simulink model "RemoteMicrogrid"  (R2025a)
settings: Solver=FixedStepAuto  StartTime=0.0  StopTime=8  FixedStep=Ts  MaxStep=1e-3  RelTol=1e-3
PreLoadFcn:
  | RemoteMicrogridInputData
undefined symbols (not defined in the file): BESS, ControlRoom, DiscIntNeverNeededParam, Grid, Load, Machine, Microgrid, MicrogridStatus, PV, relay1, T_on, Ts
libraries: ee_lib x53, fl_lib x39, eeGeneralControl x30, simulink x30, nesl_utility x26, nesl_utility_internal x19, slpidlib x7, eeTransforms x5, eeRmsMeasurement x4, eeTotalHarmonicDistorsion x4, batteryecm_lib x2, simulink_extras x2
(part 1 of 6)
CloseFcn:
  | figure1 = findobj('Type', 'figure', 'Name','h1_remote_microgrid');
  | figure2 = findobj('Type', 'figure', 'Name','h2_remote_microgrid');
  | figure3 = findobj('Type', 'figure', 'Name','h2a_remote_microgrid');
  | figure4 = findobj('Type', 'figure', 'Name','h3_remote_microgrid');
  | figure5 = findobj('Type', 'figure', 'Name','h4_remote_microgrid');
  | close(figure1);
  | close(figure2);
  | close(figure3);
  | close(figure4);
  | close(figure5);
  | clear figure1 figure2 figure3 figure4 figure5
  | clear BESS closedLoop controller currentLoopPole
  | clear fsw_V geometricMean grid Grid inverter KI_PVPLL
  | clear KP_PVPLL logsout_remote_microgrid
  | clear Microgrid PrimaryreactancePV PrimaryresistancePV
  | clear remainingPowerPerString SecondaryreactancePV
  | clear SecondaryresistancePV sensor simlog_remote_microgrid
  | clear simulation solarPanel solarPlant TransformerPrimaryVoltagePV
  | clear TransformerRatingPV TransformerSecondaryVoltagePV
  | clear Ts Ts_V Solar logsout_remote_microgrid simlog_remote_microgrid
  | clear caseNum ControlRoom Load Machine tStart tStop
  | clear transformer_lv transformer_hv transformer_VA
  | clear transformer_winding_resistance transformer_winding_lekage_reactance
  | clear transformer_zero_sequence_reactance I_max_pu Vdc C L KV_base_new
  | clear MVA_base_new z_base n_series_cell_panel n_parallel_strings_panel
  | clear n_series_panels_per_string n_parallel_strings t_sensor
  | clear Kp_ic Ki_ic Kd Kp_v Ki_v Kd_v Vdc_base
  | clear Kp_pll Ki_pll
  | clear diode_saturation_current solar_generated_current_AM
  | clear quality_factor_i quality_factor_j Solar_cell.series_resistance
  | clear parallel_resistance temp_cofficient Eg temparature_exponent_Is1
  | clear temparature_exponent_Is2 temparature_exponent_Rs temparature_exponent_Rp
  | clear measurement_temperature device_temperature
  | clear PV Solar_cell T_on
  | clear BESSCost1 BESSCost2 BESSCost3 BESSCost4 BESSCost5 BESSKVAs1 BESSKVAs2
  | clear BESSKVAs3 BESSKVAs4 BESSKVAs5 Diesel_cost_s1 Diesel_cost_s1_yr Diesel_cost_s2
  | clear Diesel_cost_s2_yr Diesel_cost_s3 Diesel_cost_s3_yr Diesel_cost_s4 Diesel_cost_s4_yr
  | clear Diesel_cost_s5 Diesel_cost_s5_yr diesel_litre_USD Diesel_loading_100percent
  | clear Diesel_loading_25percent Diesel_loading_50percent Diesel_loading_75percent
  | clear Diesel_s1 Diesel_s2 Diesel_s3 Diesel_s4 Diesel_s5 DieselKVAs1 DieselKVAs2
  | clear DieselKVAs3 DieselKVAs4 DieselKVAs5 frequencyLimit logsout1 logsout2 logsout3
  | clear logsout4 logsout_activeloss1 logsout_activeloss2 logsout_activeloss3
  | clear logsout_activeloss4 logsout_freqmax1 logsout_freqmax2 logsout_freqmax3
  | clear logsout_freqmax4 logsout_freqmin1 logsout_freqmin2 logsout_freqmin3 logsout_freqmin4
  | clear logsout_LoadTHD1 logsout_LoadTHD2 logsout_LoadTHD3 logsout_LoadTHD4
  | clear logsout_MaxLoadVoltage1 logsout_MaxLoadVoltage2 logsout_MaxLoadVoltage3
  | clear logsout_MaxLoadVoltage4 logsout_MinLoadVoltage1 logsout_MinLoadVoltage2
  | clear logsout_MinLoadVoltage3 logsout_MinLoadVoltage4 logsout_PCCTHD1 logsout_PCCTHD2
  | clear logsout_PCCTHD3 logsout_PCCTHD4 logsout_reactiveloss1 logsout_reactiveloss2
  | clear logsout_reactiveloss3 logsout_reactiveloss4 logsout_volmax1 logsout_volmax2
  | clear logsout_volmax3 logsout_volmax4 logsout_volmin1 logsout_volmin2 logsout_volmin3
  | clear logsout_volmin4 Micorgrid TotalCost1 TotalCost2 TotalCost3 TotalCost4 TotalCost5
  | clear voltageLimit xlim xticks
Description:
  | Copyright 2022 - 2023 The MathWorks, Inc.
settings Model: SimulationMode=accelerator  NumberOfSteps=10  Creator=The MathWorks, Inc.  LastModifiedBy=skota
settings SolverCC: ZeroCrossAlgorithm=Adaptive  AlgebraicLoopSolver=TrustRegion
settings DataIOCC: ExternalInput=getinputstruct(op)  InitialState=getstatestruct(op)  SaveOutput=off  DSMLogging=off  SaveTime=off  SignalLoggingName=logsout_RemoteMicrogrid  OutputTimes=[0:1.1*3*Voc/(1*2000):1.1*3*Voc/1]  ReturnWorkspaceOutputsName=simoutData
settings OptimizationCC: ReuseModelBlockBuffer=off
settings DebuggingCC: UnconnectedInputMsg=warning  UnconnectedOutputMsg=warning  UnconnectedLineMsg=warning  StateNameClashWarn=warning  ArithmeticOperatorsInVariantConditions=warning
settings HardwareCC: ProdBitPerPointer=32.0  ProdBitPerSizeT=32.0  ProdBitPerPtrDiffT=32.0  ProdWordSize=32.0  ProdHWDeviceType=Intel->x86-32 (Windows32)
settings ModelReferenceCC: PropagateSignalLabelsOutOfModel=off
settings SFSimCC: SFSimEcho=off  SimCtrlC=off  CustomCodeUndefinedFunction=UseInterfaceOnly
settings RTWCC: Toolchain=MinGW64 | gmake (64-bit Windows)  GPUComputeCapability=3.5  DLArmComputeVersion=19.05
settings CodeAppCC: StateflowObjectComments=on
settings SimscapeCC: SimscapeNominalValues="[{\"value\":\"1\",\"unit\":\"A\"},{\"value\":\"1\",\"unit\":\"bar\"},{\"value\":\"1\",\"unit\":\"cm^2\"},{\"value\":\"1\",\"unit\":\"cm^3/s\"},{\"value\":\"1\",\"unit\":\"kJ/kg\"},{\"value\":\"1\",\"unit\":\"kW\"},{\"value\":\"1\",\"unit\":\"l\"},{\"value\":\"1\",\"unit\":\"N\"},{\"value\":\"1\",\"unit\":\"N*m\"},{\"value\":\"1e3\",\"unit\":\"V\"}]"  SimscapeLogName=simlog_RemoteMicrogrid  SimscapeLogLimitData=off  SimscapeOperatingPoint=op

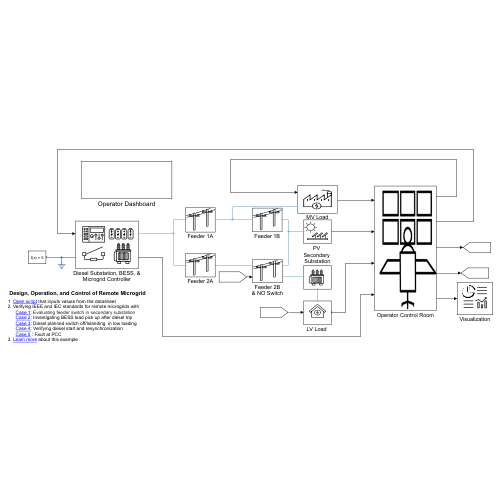
[thumbnail: Simulink's stored preview of the top-level diagram]
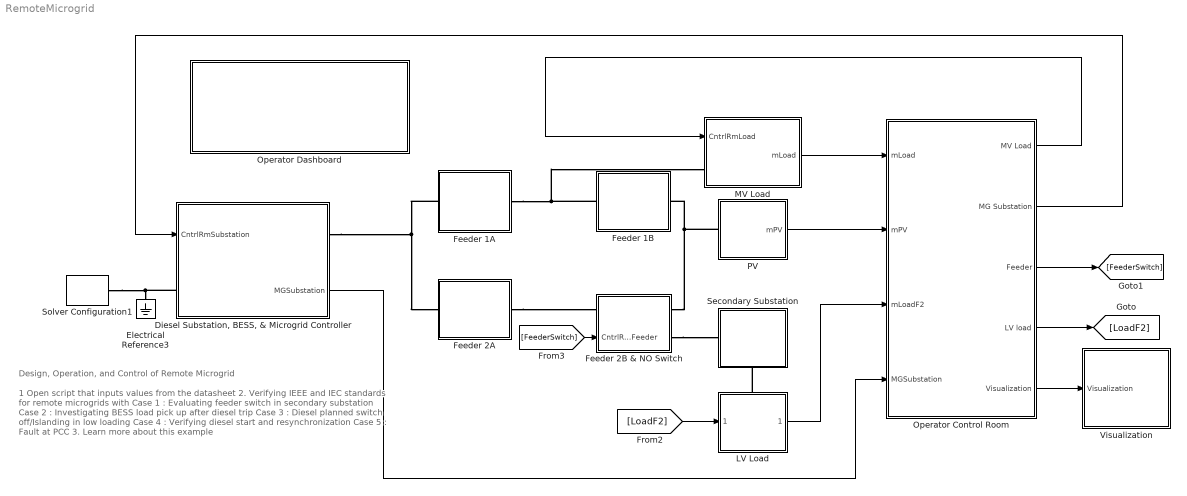
== system RemoteMicrogrid ==
  note: Design, Operation, and Control of Remote Microgrid
  note: 1 Open script that inputs values from the datasheet
      | 2. Verifying IEEE and IEC standards for remote microgrids with
      | Case 1 : Evaluating feeder switch in secondary substation
      | Case 2 : Investigating BESS load pick up after diesel trip
      | Case 3 : Diesel planned switch off/Islanding in low loading
      | Case 4 : Verifying diesel start and resynchronization
      | Case 5 : Fault at PCC
      | 3. Learn more about this example
  "Diesel Substation, BESS, & Microgrid Controller" : Subsystem
      settings: PortSchema="{\"entries\":[{\"content\":{\"sides\":[{\"content\":{\"connectorIds\":[\"In1\",\"LConn1\"]},\"type\":\"ConnectorPlacement.EquallySpacedRectSide\",\"uuid\":\"34af2ba0-e960-4f27-b72f-7309cde5bec1\"},{\"content\":{\"connectorIds\":[\"RConn1\",\"Out1\"],\"side\":\"RIGHT\"},\"type\":\"ConnectorPlacement.EquallySpacedRectSide\",\"uuid\":\"58e91d81-71e9-481c-b1fd-5cc7b2cbdd18\"},{\"content\":{\"side\":\"TOP\"},\"type\":\"ConnectorPlacement.EquallySpacedRectSide\",\"uuid\":\"32e6dd42-e4bf-406e-9b62-7b4d690f744b\"},{\"content\":{\"side\":\"BOTTOM\"},\"type\":\"ConnectorPlacement.EquallySpacedRectSide\",\"uuid\":\"17a24731-c833-4ec2-b0a2-39897b42a00f\"}]},\"type\":\"ConnectorPlacement.EquallySpacedConnector\",\"uuid\":\"86c228e9-32f4-4f18-a8a0-642828fccfbb\"}],\"packageUris\":[\"http://schema.mathworks.com/mf0/Connector/R2020b\"],\"version\":\"1.0\"}"
      mask Display: image('$imagefile'); % Use "Edit Image" on toolstrip to change.
  Electrical Reference3 : fl_lib/Electrical/Electrical Elements/Electrical Reference
  Feeder 1A : Subsystem
      mask Display: image('$imagefile'); % Use "Edit Image" on toolstrip to change.
  Feeder 1B : Subsystem
      mask Display: image('$imagefile'); % Use "Edit Image" on toolstrip to change.
  Feeder 2A : Subsystem
      mask Display: image('$imagefile'); % Use "Edit Image" on toolstrip to change.
  Feeder 2B & NO Switch : Subsystem
      settings: PortSchema="{\"entries\":[{\"content\":{\"sides\":[{\"content\":{\"connectorIds\":[\"LConn1\",\"In1\"]},\"type\":\"ConnectorPlacement.EquallySpacedRectSide\",\"uuid\":\"b1ff7143-0432-45d1-9871-6b8068209aeb\"},{\"content\":{\"connectorIds\":[\"RConn1\",\"RConn2\"],\"side\":\"RIGHT\"},\"type\":\"ConnectorPlacement.EquallySpacedRectSide\",\"uuid\":\"b6fa69ce-48c3-4fac-b04a-2b7bcdb32261\"},{\"content\":{\"side\":\"TOP\"},\"type\":\"ConnectorPlacement.EquallySpacedRectSide\",\"uuid\":\"fc1d609f-60ee-4a8a-8cbb-ab607c0d8f9d\"}]},\"type\":\"ConnectorPlacement.EquallySpacedConnector\",\"uuid\":\"7ded5dff-a611-4ac5-b5e8-d2daf052a912\"}],\"packageUris\":[\"http://schema.mathworks.com/mf0/Connector/R2020b\"],\"version\":\"1.0\"}"
      mask Display: image('$imagefile'); % Use "Edit Image" on toolstrip to change.
  "LV Load " : Subsystem
      settings: PortSchema="{\"entries\":[{\"content\":{\"sides\":[{\"content\":{\"connectorIds\":[\"In1\"]},\"type\":\"ConnectorPlacement.EquallySpacedRectSide\",\"uuid\":\"cc4763ec-9449-4f2d-b299-5261ad2f5cfe\"},{\"content\":{\"connectorIds\":[\"Out1\"],\"side\":\"RIGHT\"},\"type\":\"ConnectorPlacement.EquallySpacedRectSide\",\"uuid\":\"9da329b8-70a1-4faf-a44a-2cf8be9addec\"},{\"content\":{\"connectorIds\":[\"LConn1\"],\"side\":\"TOP\"},\"type\":\"ConnectorPlacement.EquallySpacedRectSide\",\"uuid\":\"c4abe44e-3291-4dff-9d7a-9215b8ef2faf\"}]},\"type\":\"ConnectorPlacement.EquallySpacedConnector\",\"uuid\":\"e73dbaae-f88f-4a7a-af91-27ace77c935e\"}],\"packageUris\":[\"http://schema.mathworks.com/mf0/Connector/R2020b\"],\"version\":\"1.0\"}"
      mask Display: image('$imagefile'); % Use "Edit Image" on toolstrip to change.
  MV Load : Subsystem
      mask Display: image('$imagefile'); % Use "Edit Image" on toolstrip to change.
  Operator Control Room : Subsystem
      settings: PortSchema="{\"entries\":[{\"content\":{\"sides\":[{\"content\":{\"connectorIds\":[\"Out1\",\"Out2\",\"Out3\",\"Out4\",\"Out5\"]},\"type\":\"ConnectorPlacement.EquallySpacedRectSide\",\"uuid\":\"36e3c748-e70d-4376-8c54-bee35c2cf55e\"},{\"content\":{\"connectorIds\":[\"In1\",\"In2\",\"In3\",\"In4\"],\"side\":\"RIGHT\"},\"type\":\"ConnectorPlacement.EquallySpacedRectSide\",\"uuid\":\"3af4b9ea-3351-4c6c-90c1-760bf6d2a862\"},{\"content\":{\"side\":\"TOP\"},\"type\":\"ConnectorPlacement.EquallySpacedRectSide\",\"uuid\":\"c84439f5-3dbb-4f33-afb8-95498296d6fa\"}]},\"type\":\"ConnectorPlacement.EquallySpacedConnector\",\"uuid\":\"cafa6b3a-2446-4c45-9268-4fc6f6c2350c\"}],\"packageUris\":[\"http://schema.mathworks.com/mf0/Connector/R2020b\"],\"version\":\"1.0\"}"
      mask Display: image('$imagefile'); % Use "Edit Image" on toolstrip to change.
  Operator Dashboard : Subsystem  SystemSampleTime=1e-3
  "PV " : Subsystem
      mask Display: image('$imagefile'); % Use "Edit Image" on toolstrip to change.
  Secondary Substation : Subsystem
      settings: PortSchema="{\"entries\":[{\"content\":{\"sides\":[{\"content\":{\"connectorIds\":[\"LConn1\"]},\"type\":\"ConnectorPlacement.EquallySpacedRectSide\",\"uuid\":\"e00206b4-f52b-4711-97fc-4887ea8823c3\"},{\"content\":{\"connectorIds\":[],\"side\":\"RIGHT\"},\"type\":\"ConnectorPlacement.EquallySpacedRectSide\",\"uuid\":\"71e01694-379b-4552-8103-40d657e486e9\"},{\"content\":{\"connectorIds\":[],\"side\":\"TOP\"},\"type\":\"ConnectorPlacement.EquallySpacedRectSide\",\"uuid\":\"04395bce-e736-431c-9f74-8350dc9d2f2b\"},{\"content\":{\"connectorIds\":[\"RConn1\"],\"side\":\"BOTTOM\"},\"type\":\"ConnectorPlacement.EquallySpacedRectSide\",\"uuid\":\"4a9ed1b9-5a03-4ea2-8ce4-b63f4eba4172\"}]},\"type\":\"ConnectorPlacement.EquallySpacedConnector\",\"uuid\":\"55927287-d52f-4d79-aceb-3e97c7a13d06\"}],\"packageUris\":[\"http://schema.mathworks.com/mf0/Connector/R2020b\"],\"version\":\"1.0\"}"
      mask Display: image('$imagefile'); % Use "Edit Image" on toolstrip to change.
  Solver Configuration1 : nesl_utility/Solver Configuration  PhysicalDomain=network_engine_domain  SubClassName=solver  LeftPortType=input  RightPortType=generic  Tones=[]  Harmonics=[]  SimulateNoise=off  Profile=off  UseLocalSampling=off  EnableSwitchedLinearOptims=on  FrequencyDomain=off  UseCCode=off  RelTol=0.001  AbsTol=0.001  MinStep=1e-09  ToWorkspace=off  RevertToSquareIcSolve=off  NumHomotopyIterations=100  PhasorMode=off  PhasorModeNumHarmonics=1  ConsistencySolver=NEWTON_XTOL_AFTER_FTOL  IndexReductionMethod=None  DoDC=off  ResidualTolerance=1e-09  ConsistencyTolSource=GLOBAL  ConsistencyAbsTol=0.001  ConsistencyRelTol=0.001  ConsistencyTolFactor=0.001  UseLocalSolver=on  LocalSolverChoice=NE_BACKWARD_EULER_ADVANCER  ResolveIndetEquations=off  FunctionEvalNumThread=1  LocalSolverSampleTime=Ts  DoFixedCost=on  MaxNonlinIter=1  MaxModeIter=2  ComputeImpulses=off  ImpulseIterations=2  LinearAlgebra=Sparse  LinearAlgebraNumThread=0  EquationFormulation=NE_TIME_EF  DelaysMemoryBudget=1024  AutomaticFiltering=on  FilteringTimeConstant=0.001  PartitionStorageMethod=AS_NEEDED  PartitionMemoryBudget=1024  PartitionMethod=ROBUST  MultibodyUseLocalSolver=off  MultibodyLocalSolverChoice=ODE1  MultibodyLocalSolverSampleTime=0.001
  Visualization : Subsystem
      mask Display: image('$imagefile'); % Use "Edit Image" on toolstrip to change.
  wires:
  "LV Load "/1(mLoadF2) -> Operator Control Room/3(mLoadF2)
  "PV "/1(mPV) -> Operator Control Room/2(mPV)
  [FeederSwitch] -> Feeder 2B & NO Switch/1(CntrlRmFeeder)
  MV Load/1(mLoad) -> Operator Control Room/1(mLoad)
  Operator Control Room/5(Visualization) -> Visualization/1(Visualization)
  Operator Control Room/2(MG Substation) -> "Diesel Substation, BESS, & Microgrid Controller"/1(CntrlRmSubstation)
  Operator Control Room/1(MV Load) -> MV Load/1(CntrlRmLoad)
  Operator Control Room/4(LV load) -> [LoadF2]
  Operator Control Room/3(Feeder) -> [FeederSwitch]
  [LoadF2] -> "LV Load "/1(CtrlRmF2Load)
  "Diesel Substation, BESS, & Microgrid Controller"/1(MGSubstation) -> Operator Control Room/4(MGSubstation)
  connections:
  "LV Load "/LConn1 -- Secondary Substation/RConn1
  "Diesel Substation, BESS, & Microgrid Controller"/LConn1 -- Solver Configuration1/RConn1 -- Electrical Reference3/LConn1
  "PV "/LConn1 -- Feeder 2B & NO Switch/RConn1 -- Feeder 1B/RConn1
  Feeder 1A/RConn1 -- Feeder 1B/LConn1 -- MV Load/LConn1
  Feeder 1A/LConn1 -- "Diesel Substation, BESS, & Microgrid Controller"/RConn1 -- Feeder 2A/LConn1
  Feeder 2B & NO Switch/RConn2 -- Secondary Substation/LConn1
  Feeder 2A/RConn1 -- Feeder 2B & NO Switch/LConn1

== system RemoteMicrogrid/Diesel Substation, BESS, & Microgrid Controller ==
  CntrlRmSubstation : Inport
  BESS and Controller : Subsystem
      mask Display: image('$imagefile'); % Use "Edit Image" on toolstrip to change.
  Diesel Generator : Subsystem
      mask Display: image('$imagefile'); % Use "Edit Image" on toolstrip to change.
  Microgrid Controller : Subsystem  mask{resynchronization=on, plannedIslanding=on, blackStart=off, kpPLL=Grid.PLL_Kp, kiPLL=Grid.PLL_Ki, frequencyPLL=Grid.Frequency, sampleTimePLL=Ts, pUpperLimit=Microgrid.UpperPRef, pLowerLimit=Microgrid.LowerPRef, qUpperLimit=Microgrid.UpperPRef, qLowerLimit=Microgrid.LowerPRef, gridFrequency=Grid.Frequency, resyncDelay=Microgrid.ResynchDelay, kpVoltage=Microgrid.KP_Vol_resynch, kiVoltage=Microgrid.KI_Vol_resynch, voltageThreshold=Microgrid.VoltageThreshhold, voltageDroop=Microgrid.Kdroop, kpFrequency=Microgrid.KP_fre_resynch, kiFrequency=Microgrid.KI_fre_resynch, frequencyThreshold=Microgrid.FrequencyThreshold, kpAngle=Microgrid.KP_Ang_resynch, kiAngle=Microgrid.KI_Ang_resynch, angleThreshold=Microgrid.AngleThreshold, plannedIslandingDelay=Microgrid.PlannedIslandDelay, kpActive=Microgrid.KP_P_plannedisland, kiActive=Microgrid.KI_P_plannedisland, activeThreshold=Microgrid.ZeroActivePowerThreshhold, kpReactive=Microgrid.KP_Q_plannedisland, kiReactive=Microgrid.KI_Q_plannedisland, reactiveThreshold=Microgrid.ZeroReactivePowerThreshhold, blackStartTime=100, blackStartFrequency=60, level1=0, level2=0, level3=0, delay1=0, delay2=0, delay3=0, upperVoltagelimit=1.1, lowerVoltageLimit=0.9, upperFrequencyLimit=60.6, lowerFrequencyLimit=59.4}
      mask prompts: plannedIslanding "Planned Islanding"; blackStart "Black Start"; kpPLL "Proportional Gain"; kiPLL "Integral Gain"; frequencyPLL "Grid Frequency in Hz"; sampleTimePLL "Sample Time in sec"; pUpperLimit "Upper Limit in pu"; pLowerLimit "Lower Limit in pu"; qUpperLimit "Upper Limit in pu"; qLowerLimit "Lower Limit in pu"; gridFrequency "Grid Frequency in Hz"; resyncDelay "Delay in sec"; kpVoltage "Proportional Gain"; kiVoltage "Voltage Integral Gain"; voltageThreshold "Threshold"; voltageDroop "Reactive Power Droop"; kpFrequency "Proportional Gain"; kiFrequency "Integral Gain"; frequencyThreshold "Threshold"; kpAngle "Proportional Gain"; kiAngle "Integral Gain"; angleThreshold "Threshold"; plannedIslandingDelay "Delay in sec"; kpActive "Proportional Gain"; kiActive "Integral Gain"; activeThreshold "Threshold"; kpReactive "Proportional Gain"; kiReactive "Integral Gain"; reactiveThreshold "Threshold"; blackStartTime "Black Start Time in sec"; blackStartFrequency "Reference Frequency in Hz"; level1 "Level 1 in pu"; level2 "Level 2 in pu"; level3 "Level 3 in pu"; delay1 "Delay 1 in sec"; delay2 "Delay2 in sec"; delay3 "Delay3 in sec"; upperVoltagelimit "Maximum Voltage in pu"; lowerVoltageLimit "Minimum Voltage in pu"; upperFrequencyLimit "Maximum frequency in Hz"; lowerFrequencyLimit "Minimum Frequency in Hz"
      mask init:
      | plannedIslandingBlock = [gcb,'/','Microgrid Control Functions','/','Planned Islanding'];
      | resynchBlock = [gcb,'/','Microgrid Control Functions','/','Resynchronization'];
      | blackStartBlock = [gcb,'/','Microgrid Control Functions','/','Black Start'];
      | block = {resynchBlock,plannedIslandingBlock,blackStartBlock};
      | blockEnable = {get_param(gcb,'resynchronization'),get_param(gcb,'plannedIslanding'),get_param(gcb,'blackStart')};
      | parameterIdx = {12:23,24:30,31:38};
      | % Set the 'MaskVisibilities' property for each parameters
      | cArray=cell(1,42);
      | cArray(:)={'on'};
      | for blockIdx = 1:length(block)
      |     if strcmp(blockEnable{blockIdx},'on')
      |         cArray(parameterIdx{blockIdx}) = {'on'};
      |     else
      |         cArray(parameterIdx{blockIdx}) = {'off'};
      |     end
      | end
      | set_param(gcb,'MaskVisibilities',cArray);
      mask Callback resynchronization:
      | plannedIslandingBlock = [gcb,'/','Microgrid Control Functions','/','Planned Islanding'];
      | resynchBlock = [gcb,'/','Microgrid Control Functions','/','Resynchronization'];
      | blackStartBlock = [gcb,'/','Microgrid Control Functions','/','Black Start'];
      | block = {resynchBlock,plannedIslandingBlock,blackStartBlock};
      | blockEnable = {get_param(gcb,'resynchronization'),get_param(gcb,'plannedIslanding'),get_param(gcb,'blackStart')};
      | parameterIdx = {12:23,24:30,31:38};
      | % Set the 'MaskVisibilities' property for each parameters
      | cArray=cell(1,42);
      | cArray(:)={'on'};
      | for blockIdx = 1:length(block)
      |     if strcmp(blockEnable{blockIdx},'on')
      |         cArray(parameterIdx{blockIdx}) = {'on'};
      |     else
      |         cArray(parameterIdx{blockIdx}) = {'off'};
      |     end
      | end
      | set_param(gcb,'MaskVisibilities',cArray);
      mask Callback plannedIslanding:
      | plannedIslandingBlock = [gcb,'/','Microgrid Control Functions','/','Planned Islanding'];
      | resynchBlock = [gcb,'/','Microgrid Control Functions','/','Resynchronization'];
      | blackStartBlock = [gcb,'/','Microgrid Control Functions','/','Black Start'];
      | block = {resynchBlock,plannedIslandingBlock,blackStartBlock};
      | blockEnable = {get_param(gcb,'resynchronization'),get_param(gcb,'plannedIslanding'),get_param(gcb,'blackStart')};
      | parameterIdx = {12:23,24:30,31:38};
      | % Set the 'MaskVisibilities' property for each parameters
      | cArray=cell(1,42);
      | cArray(:)={'on'};
      | for blockIdx = 1:length(block)
      |     if strcmp(blockEnable{blockIdx},'on')
      |         cArray(parameterIdx{blockIdx}) = {'on'};
      |     else
      |         cArray(parameterIdx{blockIdx}) = {'off'};
      |     end
      | end
      | set_param(gcb,'MaskVisibilities',cArray);
      mask Callback blackStart:
      | plannedIslandingBlock = [gcb,'/','Microgrid Control Functions','/','Planned Islanding'];
      | resynchBlock = [gcb,'/','Microgrid Control Functions','/','Resynchronization'];
      | blackStartBlock = [gcb,'/','Microgrid Control Functions','/','Black Start'];
      | block = {resynchBlock,plannedIslandingBlock,blackStartBlock};
      | blockEnable = {get_param(gcb,'resynchronization'),get_param(gcb,'plannedIslanding'),get_param(gcb,'blackStart')};
      | parameterIdx = {12:23,24:30,31:38};
      | % Set the 'MaskVisibilities' property for each parameters
      | cArray=cell(1,42);
      | cArray(:)={'on'};
      | for blockIdx = 1:length(block)
      |     if strcmp(blockEnable{blockIdx},'on')
      |         cArray(parameterIdx{blockIdx}) = {'on'};
      |     else
      |         cArray(parameterIdx{blockIdx}) = {'off'};
      |     end
      | end
      | set_param(gcb,'MaskVisibilities',cArray);
      mask DialogControl ParameterGroupVar Prompt: Microgrid control functions
      mask DialogControl Container22 Prompt: PLL
      mask DialogControl Container25 Prompt: General
      mask DialogControl Container23 Prompt: Reference Generation
      mask DialogControl Container27 Prompt: Active Power
      mask DialogControl Container28 Prompt: Reactive Power
      mask DialogControl Container3 Prompt: Resynchronization
      mask DialogControl Container15 Prompt: General
      mask DialogControl Container9 Prompt: Voltage
      mask DialogControl Container10 Prompt: Frequency
      mask DialogControl Container11 Prompt: Angle
      mask DialogControl Container8 Prompt: Planned Islanding
      mask DialogControl Container16 Prompt: General
      mask DialogControl Container13 Prompt: Active Power
      mask DialogControl Container14 Prompt: Reactive Power
      mask DialogControl Container17 Prompt: Black Start
      mask DialogControl Container19 Prompt: General
      mask DialogControl Container20 Prompt: Voltage Levels
      mask DialogControl Container21 Prompt: Time Delays
      mask DialogControl Container261 Prompt: Power Quality Metrics
      mask Display: image('$imagefile'); % Use "Edit Image" on toolstrip to change.
  PCC Measurements and PCC Breaker : Subsystem
      settings: PortSchema="{\"entries\":[{\"content\":{\"sides\":[{\"content\":{\"connectorIds\":[\"In1\",\"LConn1\"]},\"type\":\"ConnectorPlacement.EquallySpacedRectSide\",\"uuid\":\"04177ba8-e6a4-4482-9e4e-86e01b546ca8\"},{\"content\":{\"connectorIds\":[\"RConn1\",\"Out1\"],\"side\":\"RIGHT\"},\"type\":\"ConnectorPlacement.EquallySpacedRectSide\",\"uuid\":\"b1feeba7-b9e0-4dc8-9251-9fa4e491a467\"},{\"content\":{\"side\":\"TOP\"},\"type\":\"ConnectorPlacement.EquallySpacedRectSide\",\"uuid\":\"26b7aa1a-5290-4eee-bcf5-b11865d5ca2e\"}]},\"type\":\"ConnectorPlacement.EquallySpacedConnector\",\"uuid\":\"5841c04a-e0b1-4fd8-9efd-d8c83177b337\"}],\"packageUris\":[\"http://schema.mathworks.com/mf0/Connector/R2020b\"],\"version\":\"1.0\"}"
      mask Display: image('SImple Switch.svg');
  Transformer and Disconnectors : Subsystem
      mask Display: image('$imagefile'); % Use "Edit Image" on toolstrip to change.
  ref : PMIOPort  Side=Left
  "~ " : PMIOPort  Port=2  Side=Right
  Out Bus Element : Outport  PortName=MGSubstation  Element=mBESS
  Out Bus Element1 : Outport  PortName=MGSubstation  Element=MGController
  Out Bus Element2 : Outport  PortName=MGSubstation  Element=mPCC
  wires:
  Microgrid Controller/5(PCC BRK) -> PCC Measurements and PCC Breaker/1(Breaker)
  CntrlRmSubstation/1 -> BESS and Controller/1(CntrlRmSubstation), Microgrid Controller/1(CtrlRmSubstation)
  BESS and Controller/1(mBESS) -> Out Bus Element/1
  PCC Measurements and PCC Breaker/1(" mPCC") -> Out Bus Element2/1, Microgrid Controller/2(mPCC)
  Microgrid Controller/1(VRef) -> BESS and Controller/2(VRef)
  Microgrid Controller/2(FRef) -> BESS and Controller/3(FRef)
  Microgrid Controller/3(PQRef) -> BESS and Controller/4(PQRef)
  [MGController] -> Diesel Generator/1(MGController)
  Microgrid Controller/4(MGController) -> Out Bus Element1/1, [MGController]
  connections:
  "~ "/RConn1 -- BESS and Controller/RConn1 -- PCC Measurements and PCC Breaker/RConn1
  Transformer and Disconnectors/RConn1 -- PCC Measurements and PCC Breaker/LConn1
  Diesel Generator/RConn1 -- Transformer and Disconnectors/LConn1
  Diesel Generator/LConn1 -- ref/RConn1

== system RemoteMicrogrid/Feeder 1A ==
  "Line X/R=1.44 " : ee_lib/Passive/RLC Assemblies/RLC (Three-Phase)  port_option=ee.enum.threePhasePort.composite  component_structure=ee.enum.rlc.structure.SeriesRL  R=Microgrid.R_line Ohm  L=Microgrid.L_line H  C=1 F  R_parasitic=1e-6 Ohm  G_parasitic=1e-5 1/Ohm  IL_specify=on  IL_priority=High  IL=[0, 0, 0] A  IL_nominal_specify=off  IL_nominal_value=1  IL_nominal_unit=A  VC_specify=on  VC_priority=High  VC=[0, 0, 0] V  VC_nominal_specify=off  VC_nominal_value=1  VC_nominal_unit=V
      settings: InternalSimscapePortConfiguration="{\"Bottom\":[],\"Left\":[{\"id\":\"N1\",\"label\":\"~1\",\"type\":\"foundation.electrical.three_phase\"}],\"Right\":[{\"id\":\"N2\",\"label\":\"~2\",\"type\":\"foundation.electrical.three_phase\"}],\"Top\":[]}"
  Conn1 : PMIOPort  Side=Right
  Conn2 : PMIOPort  Port=2  Side=Left
  connections:
  "Line X/R=1.44 "/RConn1 -- Conn1/RConn1
  "Line X/R=1.44 "/LConn1 -- Conn2/RConn1

== system RemoteMicrogrid/Feeder 1B ==
  Line X/R=1.44 : ee_lib/Passive/RLC Assemblies/RLC (Three-Phase)  port_option=ee.enum.threePhasePort.composite  component_structure=ee.enum.rlc.structure.SeriesRL  R=Microgrid.R_line Ohm  L=Microgrid.L_line H  C=1 F  R_parasitic=1e-6 Ohm  G_parasitic=1e-5 1/Ohm  IL_specify=on  IL_priority=High  IL=[0, 0, 0] A  IL_nominal_specify=off  IL_nominal_value=1  IL_nominal_unit=A  VC_specify=on  VC_priority=High  VC=[0, 0, 0] V  VC_nominal_specify=off  VC_nominal_value=1  VC_nominal_unit=V
      settings: InternalSimscapePortConfiguration="{\"Bottom\":[],\"Left\":[{\"id\":\"N1\",\"label\":\"~1\",\"type\":\"foundation.electrical.three_phase\"}],\"Right\":[{\"id\":\"N2\",\"label\":\"~2\",\"type\":\"foundation.electrical.three_phase\"}],\"Top\":[]}"
  Conn1 : PMIOPort  Side=Left
  Conn2 : PMIOPort  Port=2  Side=Right
  connections:
  Line X/R=1.44/LConn1 -- Conn1/RConn1
  Conn2/RConn1 -- Line X/R=1.44/RConn1

== system RemoteMicrogrid/Feeder 2A ==
  "Line X/R=1.44  " : ee_lib/Passive/RLC Assemblies/RLC (Three-Phase)  port_option=ee.enum.threePhasePort.composite  component_structure=ee.enum.rlc.structure.SeriesRL  R=Microgrid.R_line Ohm  L=Microgrid.L_line H  C=1 F  R_parasitic=1e-6 Ohm  G_parasitic=1e-5 1/Ohm  IL_specify=on  IL_priority=High  IL=[0, 0, 0] A  IL_nominal_specify=off  IL_nominal_value=1  IL_nominal_unit=A  VC_specify=on  VC_priority=High  VC=[0, 0, 0] V  VC_nominal_specify=off  VC_nominal_value=1  VC_nominal_unit=V
      settings: InternalSimscapePortConfiguration="{\"Bottom\":[],\"Left\":[{\"id\":\"N1\",\"label\":\"~1\",\"type\":\"foundation.electrical.three_phase\"}],\"Right\":[{\"id\":\"N2\",\"label\":\"~2\",\"type\":\"foundation.electrical.three_phase\"}],\"Top\":[]}"
  Conn2 : PMIOPort  Side=Left
  Conn1 : PMIOPort  Port=2  Side=Right
  connections:
  Conn2/RConn1 -- "Line X/R=1.44  "/LConn1
  Conn1/RConn1 -- "Line X/R=1.44  "/RConn1

== system RemoteMicrogrid/Feeder 2B & NO Switch ==
  Bus Element In2 : Inport  PortName=CntrlRmFeeder  Element=FeederSwitch
  " Line X/R=1.44 " : ee_lib/Passive/RLC Assemblies/RLC (Three-Phase)  port_option=ee.enum.threePhasePort.composite  component_structure=ee.enum.rlc.structure.SeriesRL  R=Microgrid.R_line Ohm  L=Microgrid.L_line H  C=1 F  R_parasitic=1e-6 Ohm  G_parasitic=1e-5 1/Ohm  IL_specify=on  IL_priority=High  IL=[0, 0, 0] A  IL_nominal_specify=off  IL_nominal_value=1  IL_nominal_unit=A  VC_specify=on  VC_priority=High  VC=[0, 0, 0] V  VC_nominal_specify=off  VC_nominal_value=1  VC_nominal_unit=V
      settings: InternalSimscapePortConfiguration="{\"Bottom\":[],\"Left\":[{\"id\":\"N1\",\"label\":\"~1\",\"type\":\"foundation.electrical.three_phase\"}],\"Right\":[{\"id\":\"N2\",\"label\":\"~2\",\"type\":\"foundation.electrical.three_phase\"}],\"Top\":[]}"
  " Line X/R=1.44 1" : ee_lib/Passive/RLC Assemblies/RLC (Three-Phase)  port_option=ee.enum.threePhasePort.composite  component_structure=ee.enum.rlc.structure.SeriesRL  R=Microgrid.R_line Ohm  L=Microgrid.L_line H  C=1 F  R_parasitic=1e-6 Ohm  G_parasitic=1e-5 1/Ohm  IL_specify=on  IL_priority=High  IL=[0, 0, 0] A  IL_nominal_specify=off  IL_nominal_value=1  IL_nominal_unit=A  VC_specify=on  VC_priority=High  VC=[0, 0, 0] V  VC_nominal_specify=off  VC_nominal_value=1  VC_nominal_unit=V
      settings: InternalSimscapePortConfiguration="{\"Bottom\":[],\"Left\":[{\"id\":\"N1\",\"label\":\"~1\",\"type\":\"foundation.electrical.three_phase\"}],\"Right\":[{\"id\":\"N2\",\"label\":\"~2\",\"type\":\"foundation.electrical.three_phase\"}],\"Top\":[]}"
  Circuit Breaker : Subsystem
  Circuit Breaker1 : Subsystem
  Subsystem : Subsystem
  Conn2 : PMIOPort  Side=Left
  Feeder1BRK : PMIOPort  Port=2  Side=Right
  Feeder2BRK : PMIOPort  Port=3  Side=Right
  wires:
  Bus Element In2/1 -> Subsystem/1(ControlRoom)
  Subsystem/2(Output1) -> Circuit Breaker/1(BRK)
  Subsystem/1(Output) -> Circuit Breaker1/1(BRK)
  connections:
  Circuit Breaker1/LConn1 -- " Line X/R=1.44 "/RConn1
  " Line X/R=1.44 1"/LConn1 -- Feeder2BRK/RConn1
  Circuit Breaker/LConn1 -- Conn2/RConn1
  " Line X/R=1.44 1"/RConn1 -- Circuit Breaker/RConn1 -- " Line X/R=1.44 "/LConn1
  Circuit Breaker1/RConn1 -- Feeder1BRK/RConn1

== system RemoteMicrogrid/LV Load  ==
  Bus Element In3 : Inport  PortName=CtrlRmF2Load  Element=Load2BControl
  Bus Element In1 : Inport  PortName=CtrlRmF2Load  Element=Load2AControl
  Circuit Breaker : Subsystem
  Circuit Breaker 1 : Subsystem
  Electrical Reference2 : fl_lib/Electrical/Electrical Elements/Electrical Reference
  Electrical Reference5 : fl_lib/Electrical/Electrical Elements/Electrical Reference
  Load Measurements1 : Subsystem
  Switchable 10 kW 480 Vrms 60 Hz : ee_lib/Passive/RLC Assemblies/Wye-Connected Load  port_option=ee.enum.threePhasePort.composite  parameterization=ee.enum.rlc.parameterization.ratedpower  component_structure=ee.enum.rlc.structure.C  component_structure_PQ=ee.enum.rlc.structure.SeriesRL  R=1 Ohm  L=0.001 H  C=1e-6 F  VRated=Microgrid.LVVoltage V  FRated=Microgrid.Frequency Hz  P=Microgrid.P_LoadF2B W  Qpos=Microgrid.Q_LoadF2B A*V  Qneg=-3000 A*V  R_parasitic=1e-6 Ohm  G_parasitic=1e-6 1/Ohm  R_parasitic_PQ=1e-6 Ohm  G_parasitic_PQ=1e-6 1/Ohm  Vmag0=0 V  Vang0=0 deg  Freq0=Microgrid.Frequency Hz  IL_specify=on  IL_priority=High  IL=[ 0 0 0 ] A  IL_nominal_specify=off  IL_nominal_value=1  IL_nominal_unit=A  VC_specify=on  VC_priority=High  VC=[ 0 0 0 ] V  VC_nominal_specify=off  VC_nominal_value=1  VC_nominal_unit=V
  Switchable 25 kW 480 Vrms 60 Hz : ee_lib/Passive/RLC Assemblies/Wye-Connected Load  port_option=ee.enum.threePhasePort.composite  parameterization=ee.enum.rlc.parameterization.ratedpower  component_structure=ee.enum.rlc.structure.C  component_structure_PQ=ee.enum.rlc.structure.SeriesRL  R=1 Ohm  L=0.001 H  C=1e-6 F  VRated=Microgrid.LVVoltage V  FRated=Microgrid.Frequency Hz  P=Microgrid.P_LoadF2A W  Qpos=Microgrid.Q_LoadF2A A*V  Qneg=-3000 A*V  R_parasitic=1e-6 Ohm  G_parasitic=1e-6 1/Ohm  R_parasitic_PQ=1e-6 Ohm  G_parasitic_PQ=1e-6 1/Ohm  Vmag0=0 V  Vang0=0 deg  Freq0=Microgrid.Frequency Hz  IL_specify=on  IL_priority=High  IL=[ 0 0 0 ] A  IL_nominal_specify=off  IL_nominal_value=1  IL_nominal_unit=A  VC_specify=on  VC_priority=High  VC=[ 0 0 0 ] V  VC_nominal_specify=off  VC_nominal_value=1  VC_nominal_unit=V
  ~ : PMIOPort  Side=Left
  mLoadF2 : Outport
  wires:
  Load Measurements1/1(mLoadF2) -> mLoadF2/1
  Bus Element In3/1 -> Circuit Breaker 1/1(BRK)
  Bus Element In1/1 -> Circuit Breaker/1(BRK)
  connections:
  Electrical Reference2/LConn1 -- Switchable 25 kW 480 Vrms 60 Hz/RConn1
  ~/RConn1 -- Load Measurements1/LConn1
  Circuit Breaker/RConn1 -- Switchable 25 kW 480 Vrms 60 Hz/LConn1
  Switchable 10 kW 480 Vrms 60 Hz/RConn1 -- Electrical Reference5/LConn1
  Load Measurements1/RConn1 -- Circuit Breaker/LConn1 -- Circuit Breaker 1/LConn1
  Circuit Breaker 1/RConn1 -- Switchable 10 kW 480 Vrms 60 Hz/LConn1

== system RemoteMicrogrid/MV Load ==
  Bus Element In3 : Inport  PortName=CntrlRmLoad  Element=Load2Control
  Bus Element In1 : Inport  PortName=CntrlRmLoad  Element=Load1Control
  Circuit Breaker : Subsystem
  Circuit Breaker1 : Subsystem
  Electrical Reference2 : fl_lib/Electrical/Electrical Elements/Electrical Reference
  Electrical Reference5 : fl_lib/Electrical/Electrical Elements/Electrical Reference
  Load Measurements1 : Subsystem
  Switchable 115 kW 4160 Vrms 60 Hz : ee_lib/Passive/RLC Assemblies/Wye-Connected Load  port_option=ee.enum.threePhasePort.composite  parameterization=ee.enum.rlc.parameterization.ratedpower  component_structure=ee.enum.rlc.structure.C  component_structure_PQ=ee.enum.rlc.structure.SeriesRL  R=1 Ohm  L=0.001 H  C=1e-6 F  VRated=Microgrid.Voltage V  FRated=Microgrid.Frequency Hz  P=Microgrid.P_LoadF1A W  Qpos=Microgrid.Q_LoadF1A A*V  Qneg=-3000 A*V  R_parasitic=1e-6 Ohm  G_parasitic=1e-6 1/Ohm  R_parasitic_PQ=1e-6 Ohm  G_parasitic_PQ=1e-6 1/Ohm  Vmag0=0 V  Vang0=0 deg  Freq0=Microgrid.Frequency Hz  IL_specify=on  IL_priority=High  IL=[ 0 0 0 ] A  IL_nominal_specify=off  IL_nominal_value=1  IL_nominal_unit=A  VC_specify=on  VC_priority=High  VC=[ 0 0 0 ] V  VC_nominal_specify=off  VC_nominal_value=1  VC_nominal_unit=V
  Switchable 30 kW 4160 Vrms 60 Hz1 : ee_lib/Passive/RLC Assemblies/Wye-Connected Load  port_option=ee.enum.threePhasePort.composite  parameterization=ee.enum.rlc.parameterization.ratedpower  component_structure=ee.enum.rlc.structure.C  component_structure_PQ=ee.enum.rlc.structure.SeriesRL  R=1 Ohm  L=0.001 H  C=1e-6 F  VRated=Microgrid.Voltage V  FRated=Microgrid.Frequency Hz  P=Microgrid.P_LoadF1B W  Qpos=Microgrid.Q_LoadF1B A*V  Qneg=-3000 A*V  R_parasitic=1e-6 Ohm  G_parasitic=1e-6 1/Ohm  R_parasitic_PQ=1e-6 Ohm  G_parasitic_PQ=1e-6 1/Ohm  Vmag0=0 V  Vang0=0 deg  Freq0=Microgrid.Frequency Hz  IL_specify=on  IL_priority=High  IL=[ 0 0 0 ] A  IL_nominal_specify=off  IL_nominal_value=1  IL_nominal_unit=A  VC_specify=on  VC_priority=High  VC=[ 0 0 0 ] V  VC_nominal_specify=off  VC_nominal_value=1  VC_nominal_unit=V
  ~ : PMIOPort  Side=Left
  mLoad : Outport
  wires:
  Load Measurements1/1(mLoad) -> mLoad/1
  Bus Element In1/1 -> Circuit Breaker1/1(BRK)
  Bus Element In3/1 -> Circuit Breaker/1(BRK)
  connections:
  Switchable 30 kW 4160 Vrms 60 Hz1/RConn1 -- Electrical Reference5/LConn1
  Circuit Breaker/RConn1 -- Switchable 30 kW 4160 Vrms 60 Hz1/LConn1
  Circuit Breaker1/RConn1 -- Switchable 115 kW 4160 Vrms 60 Hz/LConn1
  ~/RConn1 -- Load Measurements1/LConn1
  Load Measurements1/RConn1 -- Circuit Breaker/LConn1 -- Circuit Breaker1/LConn1
  Electrical Reference2/LConn1 -- Switchable 115 kW 4160 Vrms 60 Hz/RConn1

== system RemoteMicrogrid/Operator Control Room ==
  mLoad : Inport
  mPV : Inport  Port=2
  mLoadF2 : Inport  Port=3
  MGSubstation : Inport  Port=4
  Load Control : Subsystem
  "Measurements and Visualizations " : Subsystem
  Microgrid Control : Subsystem
  Performance and Power Quality : Subsystem  SystemSampleTime=1e-3
  MV Load : Outport
  MG Substation : Outport  Port=2
  Feeder : Outport  Port=3
  LV load : Outport  Port=4
  Visualization : Outport  Port=5
  wires:
  mPV/1 -> "Measurements and Visualizations "/2(mPV)  "mPV"
  mLoad/1 -> "Measurements and Visualizations "/3(mLoad)  "mLoad"
  mLoadF2/1 -> "Measurements and Visualizations "/4(mLoadF2)
  "Measurements and Visualizations "/1(Visualization) -> Visualization/1, Performance and Power Quality/1(Visualization)  "Visualization"
  Microgrid Control/1(CtrlRmSubstation) -> MG Substation/1  "CtrlRmSubstation"
  Microgrid Control/2(CtrlRmFeeder) -> Feeder/1  "CtrlRMFeeder"
  Load Control/1(CtrlRmLoad) -> MV Load/1  "CtrlRmLoad"
  Load Control/2(CtrlRmF2Load) -> LV load/1  "CtrlRmF2Load"
  MGSubstation/1 -> Microgrid Control/1(MG Substation), Load Control/1(MGSubstation), "Measurements and Visualizations "/1(MGSubstation)

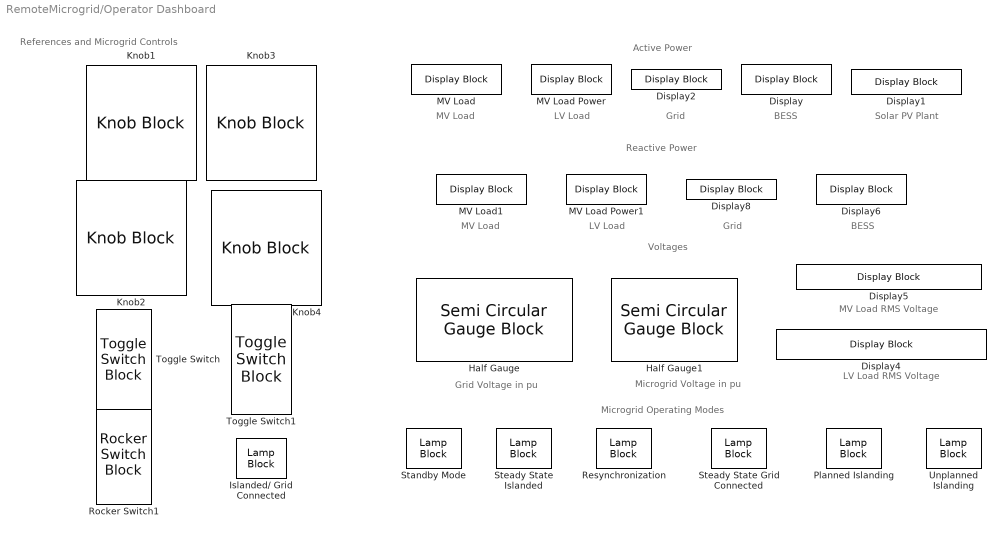
== system RemoteMicrogrid/Operator Dashboard ==
  note: Grid Voltage in pu
  note: Voltages
  note: Active Power
  note: MV Load RMS Voltage
  note: Solar PV Plant
  note: BESS
  note: Grid
  note: LV Load
  note: MV Load
  note: References and Microgrid Controls
  note: LV Load RMS Voltage
  note: Grid
  note: LV Load
  note: BESS
  note: MV Load
  note: Reactive Power
  note: Microgrid Operating Modes
  note: Microgrid Voltage in pu
  Display{,1..2,4..6,8} (7 alike) : DisplayBlock  LabelPosition=Hide  Transparency=1  GridColor=[0.502, 0.502, 0.502]
  Half Gauge : SemiCircularGaugeBlock  ScaleMax=2  FontColor=[0.0, 0.0, 0.0]
  Half Gauge1 : SemiCircularGaugeBlock  ScaleMax=2  FontColor=[0.0, 0.0, 0.0]
  Islanded/ Grid Connected : LampBlock  LabelPosition=Hide  DefaultColor=[192.0, 192.0, 192.0]
  Knob1 : KnobBlock  ScaleMax=1
  Knob2 : KnobBlock  ScaleMax=1
  Knob3 : KnobBlock  ScaleMax=1
  Knob4 : KnobBlock  ScaleMin=50  ScaleMax=70
  MV Load : DisplayBlock  LabelPosition=Hide  Transparency=1  GridColor=[0.502, 0.502, 0.502]
  MV Load Power : DisplayBlock  LabelPosition=Hide  Transparency=1  GridColor=[0.502, 0.502, 0.502]
  MV Load Power1 : DisplayBlock  LabelPosition=Hide  Transparency=1  GridColor=[0.502, 0.502, 0.502]
  MV Load1 : DisplayBlock  LabelPosition=Hide  Transparency=1  GridColor=[0.502, 0.502, 0.502]
  Planned Islanding : LampBlock  DefaultColor=[192.0, 192.0, 192.0]
  Resynchronization : LampBlock  DefaultColor=[192.0, 192.0, 192.0]
  Rocker Switch1 : RockerSwitchBlock
  Standby Mode : LampBlock  DefaultColor=[192.0, 192.0, 192.0]
  Steady State Grid Connected : LampBlock  DefaultColor=[192.0, 192.0, 192.0]
  Steady State Islanded : LampBlock  DefaultColor=[192.0, 192.0, 192.0]
  Toggle Switch : ToggleSwitchBlock
  Toggle Switch1 : ToggleSwitchBlock
  Unplanned Islanding : LampBlock  DefaultColor=[192.0, 192.0, 192.0]

== system RemoteMicrogrid/PV  ==
  30 kW PV : Subsystem
      settings: PortSchema="{\"entries\":[{\"content\":{\"sides\":[{\"content\":{\"connectorIds\":[\"Out1\",\"In1\",\"LConn1\"]},\"type\":\"ConnectorPlacement.EquallySpacedRectSide\",\"uuid\":\"cc4763ec-9449-4f2d-b299-5261ad2f5cfe\"},{\"content\":{\"connectorIds\":[],\"side\":\"RIGHT\"},\"type\":\"ConnectorPlacement.EquallySpacedRectSide\",\"uuid\":\"9da329b8-70a1-4faf-a44a-2cf8be9addec\"},{\"content\":{\"connectorIds\":[],\"side\":\"TOP\"},\"type\":\"ConnectorPlacement.EquallySpacedRectSide\",\"uuid\":\"c4abe44e-3291-4dff-9d7a-9215b8ef2faf\"}]},\"type\":\"ConnectorPlacement.EquallySpacedConnector\",\"uuid\":\"e73dbaae-f88f-4a7a-af91-27ace77c935e\"}],\"packageUris\":[\"http://schema.mathworks.com/mf0/Connector/R2020b\"],\"version\":\"1.0\"}"
  415 V/ 4.16 kV : ee_lib/Passive/Transformers/Two-Winding Transformer (Three-Phase)  SRated=PV.transformer_VA A*V  FRated=Grid.Frequency Hz  Winding1Connection=ee.enum.windingconnection.Yg  VRated1=PV.transformer_hv V  Winding2Connection=ee.enum.windingconnection.Yn  VRated2=PV.transformer_lv V  CoreType=ee.enum.coretype.threelimb  pu_Rw1=PV.transformer_winding_resistance/2  pu_Rw2=PV.transformer_winding_resistance/2  leakage_reactance_option=ee.enum.transformer_leakage.include  pu_Xl1=PV.transformer_winding_lekage_reactance/2  pu_Xl2=PV.transformer_winding_lekage_reactance/2  magnetizing_resistance_option=ee.enum.transformer_magnetizingResistance.exclude  pu_Rm=500  magnetizing_reactance_option=ee.enum.transformer_magnetizingReactance.exclude  saturation_option=ee.enum.transformer_saturation.exclude  pu_Xm=500  current_data=[0, .002, 1, 2]  magnetic_flux_data=[0, 1.2, 1.5, 1.51]  pu_X0=PV.transformer_zero_sequence_reactance  i1_specify=off  i1_priority=None  i1=[0, 0, 0] A  i1_nominal_specify=off  i1_nominal_value=1  i1_nominal_unit=A  i2_specify=off  i2_priority=None  i2=[0, 0, 0] A  i2_nominal_specify=off  i2_nominal_value=1  i2_nominal_unit=A  phi_specify=off  phi_priority=None  phi=[0, 0, 0]  phi_nominal_specify=off  phi_nominal_value=1  phi_nominal_unit=1  power_dissipated_specify=off  power_dissipated_priority=None  power_dissipated=0 W  power_dissipated_nominal_specify=off  power_dissipated_nominal_value=1  power_dissipated_nominal_unit=W
      settings: InternalSimscapePortConfiguration="{\"Bottom\":[],\"Left\":[{\"id\":\"N1\",\"label\":\"~1\",\"type\":\"foundation.electrical.three_phase\"}],\"Right\":[{\"id\":\"N2\",\"label\":\"~2\",\"type\":\"foundation.electrical.three_phase\"},{\"id\":\"n2\",\"label\":\"n2\",\"type\":\"foundation.electrical.electrical\"}],\"Top\":[]}"
  Bus Creator : BusCreator  Inputs=3
  Bus Creator1 : BusCreator  Inputs=2
  Current and Voltage Sensor (Three-Phase)5 : ee_lib/Sensors & Transducers/Current and Voltage Sensor (Three-Phase)  vMeasurementType=ee.enum.vmeasurement.lg  outputUnit=ee.enum.unit.pu  SRated=PV.MVA_base_new A*V  VRated=PV.KV_base_new V  I_specify=off  I_priority=None  I=[0, 0, 0] A  I_nominal_specify=off  I_nominal_value=1  I_nominal_unit=A  V_specify=off  V_priority=None  V=[0, 0, 0] V  V_nominal_specify=off  V_nominal_value=1  V_nominal_unit=V
      settings: InternalSimscapePortConfiguration="{\"Bottom\":[],\"Left\":[{\"id\":\"N1\",\"label\":\"~1\",\"type\":\"foundation.electrical.three_phase\"}],\"Right\":[{\"id\":\"V_output\",\"label\":\"V\",\"type\":\"output\"},{\"id\":\"I_output\",\"label\":\"I\",\"type\":\"output\"},{\"id\":\"N2\",\"label\":\"~2\",\"type\":\"foundation.electrical.three_phase\"}],\"Top\":[]}"
  Electrical Reference8 : fl_lib/Electrical/Electrical Elements/Electrical Reference
  PLL & Measurements : Subsystem
      settings: PortSchema="{\"entries\":[{\"content\":{\"sides\":[{\"content\":{\"connectorIds\":[\"Out1\",\"In1\"]},\"type\":\"ConnectorPlacement.EquallySpacedRectSide\",\"uuid\":\"76485780-20fe-4fcf-8224-69648da6ed2a\"},{\"content\":{\"connectorIds\":[],\"side\":\"RIGHT\"},\"type\":\"ConnectorPlacement.EquallySpacedRectSide\",\"uuid\":\"f19a6390-e634-42c7-8d46-4cd80cbab182\"},{\"content\":{\"connectorIds\":[],\"side\":\"TOP\"},\"type\":\"ConnectorPlacement.EquallySpacedRectSide\",\"uuid\":\"87682f72-1844-428e-be70-ad7ca3191ee3\"}]},\"type\":\"ConnectorPlacement.EquallySpacedConnector\",\"uuid\":\"f2136b07-48ec-402b-adb3-18c0bac2157c\"}],\"packageUris\":[\"http://schema.mathworks.com/mf0/Connector/R2020b\"],\"version\":\"1.0\"}"
  PS-Simulink Converter1 : nesl_utility/PS-Simulink Converter  PhysicalDomain=network_engine_domain  SubClassName=ps_output  LeftPortType=input  RightPortType=output  PseudoPeriodic=off  Frequencies=[]  VectorFormat=inherit  Unit=inherit  AffineConversion=off
  PS-Simulink Converter2 : nesl_utility/PS-Simulink Converter  PhysicalDomain=network_engine_domain  SubClassName=ps_output  LeftPortType=input  RightPortType=output  PseudoPeriodic=off  Frequencies=[]  VectorFormat=inherit  Unit=inherit  AffineConversion=off
  ~ : PMIOPort  Side=Left
  mPV : Outport
  wires:
  PS-Simulink Converter2/1 -> Bus Creator1/1, PLL & Measurements/1(V)  "Va"
  PLL & Measurements/1(PV) -> Bus Creator/2, 30 kW PV/1(PV)  "PV voltage"
  30 kW PV/1(PV power) -> Bus Creator/1  "PV power"
  Bus Creator/1 -> mPV/1
  PS-Simulink Converter1/1 -> Bus Creator1/2  "Ia"
  Bus Creator1/1 -> Bus Creator/3  "PV ac"
  connections:
  Electrical Reference8/LConn1 -- 415 V/ 4.16 kV/RConn2
  ~/RConn1 -- 415 V/ 4.16 kV/LConn1
  30 kW PV/LConn1 -- Current and Voltage Sensor (Three-Phase)5/LConn1
  PS-Simulink Converter2/LConn1 -- Current and Voltage Sensor (Three-Phase)5/RConn1
  Current and Voltage Sensor (Three-Phase)5/RConn2 -- PS-Simulink Converter1/LConn1
  415 V/ 4.16 kV/RConn1 -- Current and Voltage Sensor (Three-Phase)5/RConn3

== system RemoteMicrogrid/Secondary Substation ==
  Two-Winding Transformer (Three-Phase)1 : ee_lib/Passive/Transformers/Two-Winding Transformer (Three-Phase)  SRated=Microgrid.LVLoadTransformerRating A*V  FRated=Grid.Frequency Hz  Winding1Connection=ee.enum.windingconnection.Y  VRated1=Microgrid.LVLoadTransformerPrimaryRating V  Winding2Connection=ee.enum.windingconnection.Y  VRated2=Microgrid.LVLoadTransformerSecondaryRating V  CoreType=ee.enum.coretype.threelimb  pu_Rw1=Grid.Primaryresistance  pu_Rw2=Grid.Primaryreactance  leakage_reactance_option=ee.enum.transformer_leakage.include  pu_Xl1=Grid.Secondaryresistance  pu_Xl2=Grid.Secondaryreactance  magnetizing_resistance_option=ee.enum.transformer_magnetizingResistance.include  pu_Rm=500  magnetizing_reactance_option=ee.enum.transformer_magnetizingReactance.include  saturation_option=ee.enum.transformer_saturation.exclude  pu_Xm=500  current_data=[0, .002, 1, 2]  magnetic_flux_data=[0, 1.2, 1.5, 1.51]  pu_X0=0.5  i1_specify=on  i1_priority=None  i1=[0, 0, 0] A  i1_nominal_specify=off  i1_nominal_value=1  i1_nominal_unit=A  i2_specify=on  i2_priority=None  i2=[0, 0, 0] A  i2_nominal_specify=off  i2_nominal_value=1  i2_nominal_unit=A  phi_specify=off  phi_priority=None  phi=[0, 0, 0]  phi_nominal_specify=off  phi_nominal_value=1  phi_nominal_unit=1  power_dissipated_specify=off  power_dissipated_priority=None  power_dissipated=0 W  power_dissipated_nominal_specify=off  power_dissipated_nominal_value=1  power_dissipated_nominal_unit=W
      settings: InternalSimscapePortConfiguration="{\"Bottom\":[],\"Left\":[{\"id\":\"N1\",\"label\":\"~1\",\"type\":\"foundation.electrical.three_phase\"}],\"Right\":[{\"id\":\"N2\",\"label\":\"~2\",\"type\":\"foundation.electrical.three_phase\"}],\"Top\":[]}"
  "~ " : PMIOPort  Side=Left
  ~ : PMIOPort  Port=2  Side=Right
  connections:
  Two-Winding Transformer (Three-Phase)1/RConn1 -- ~/RConn1
  "~ "/RConn1 -- Two-Winding Transformer (Three-Phase)1/LConn1

== system RemoteMicrogrid/Visualization ==
  Bus Element In5 : Inport  PortName=Visualization  Element=BESS.activePower
  Bus Element In9 : Inport  PortName=Visualization  Element=BESS.reactivePower
  Bus Element In4 : Inport  PortName=Visualization  Element=Diesel.activePower
  Bus Element In8 : Inport  PortName=Visualization  Element=Diesel.reactivePower
  Bus Element In6 : Inport  PortName=Visualization  Element=Load.activePower
  Bus Element In10 : Inport  PortName=Visualization  Element=Load.reactivePower
  Bus Element In7 : Inport  PortName=Visualization  Element=PV.activePower
  Bus Creator : BusCreator  Inputs=4
  Bus Creator1 : BusCreator  Inputs=3
  Power  Measurements : Scope  NumInputPorts=2
      settings: Title=Active Power (kW)  ActiveDisplayYMinimum=-50.35152  ActiveDisplayYMaximum=218.62393  DataLoggingDecimation=10  DataLoggingVariableName=ScopeData3
  wires:
  Bus Element In5/1 -> Bus Creator/2  "BESS Active Power"
  Bus Element In9/1 -> Bus Creator1/2  "BESS Reactive Power"
  Bus Element In6/1 -> Bus Creator/3  "Load Active Power"
  Bus Element In8/1 -> Bus Creator1/1  "Grid Reactive Power"
  Bus Element In10/1 -> Bus Creator1/3  "Load Reactive Power"
  Bus Creator/1 -> Power  Measurements/1
  Bus Element In4/1 -> Bus Creator/1  "Diesel Active Power"
  Bus Creator1/1 -> Power  Measurements/2
  Bus Element In7/1 -> Bus Creator/4  "PV Active Power"

== system RemoteMicrogrid/Diesel Substation, BESS, & Microgrid Controller/BESS and Controller ==
  CntrlRmSubstation : Inport
  VRef : Inport  Port=2
  FRef : Inport  Port=3
  PQRef : Inport  Port=4
  BESS : Subsystem
  BESS Control : Subsystem  mask{Kp_P=BESS.Kp_P, Ki_P=BESS.Ki_P, Kp_Q=BESS.Kp_Q, Ki_Q=BESS.Ki_Q, Kp_vd=BESS.Kp_vd, Ki_vd=BESS.Ki_vd, Kp_vq=BESS.Kp_vq, Ki_vq=BESS.Ki_vq}
      mask prompts: Kp_P "Active power tracking proportional gain"; Ki_P "Active power tracking integral gain"; Kp_Q "Reactive power tracking proportional gain"; Ki_Q "Reactive power tracking integral gain"; Kp_vd "d axis voltage controller proportional gain"; Ki_vd "d axis voltage controller integral gain"; Kp_vq "q axis voltage controller proportional gain"; Ki_vq "q axis voltage controller integral gain"
  "BESS Converter Measurement " : Subsystem
  BESS Output Filter and Transformer : Subsystem
  ~ : PMIOPort  Side=Right
  mBESS : Outport
  wires:
  "BESS Converter Measurement "/1(mBESS) -> BESS Control/1(mBESS), mBESS/1  "mBESS"
  VRef/1 -> BESS Control/2(VRef)
  FRef/1 -> BESS Control/3(FRef)
  CntrlRmSubstation/1 -> BESS Control/5(CntrlRmSubstation)
  PQRef/1 -> BESS Control/4(PQref)
  connections:
  "BESS Converter Measurement "/LConn1 -- BESS Output Filter and Transformer/RConn1
  BESS Control/RConn1 -- BESS/LConn1
  BESS/LConn2 -- BESS Output Filter and Transformer/LConn1
  "BESS Converter Measurement "/RConn1 -- ~/RConn1
